simulink model "psbcompensated"  (Simulink 6.0)
settings: Solver=ode15s  SolverMode=SingleTasking  StartTime=0.0  StopTime=0.4  RelTol=1e-4
InitFcn:
  | powericon('psbinitsys',bdroot);
libraries: powerlib2 x35
settings Model: Creator=patrice  LastModifiedBy=batserve  ExtModeTrigMode=oneshot  ExtModeArmWhenConnect=off  ExtModeAutoUpdateStatusClock=off
settings DataIOCC: ExternalInput=[]  LimitDataPoints=off  SaveOutput=off  SignalLoggingName=sigsOut
settings OptimizationCC: BlockReduction=off  BooleanDataType=off
settings DebuggingCC: AlgebraicLoopMsg=none  CheckExecutionContextPreStartOutputMsg=on  CheckExecutionContextRuntimeOutputMsg=on  SolverPrmCheckMsg=none
settings HardwareCC: TargetUnknown=on
settings RTWCC: TemplateMakefile=grt_unix.tmf

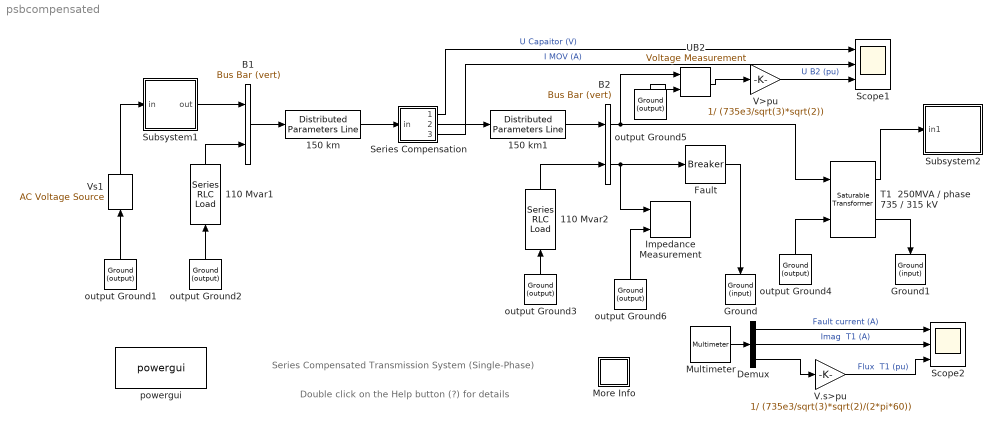
== system psbcompensated ==
  note: Series Compensated Transmission System
      | (Single-Phase)
  note: Double click on the Help button (?) for details
  110 Mvar1 : powerlib2/Elements/Series RLC Load  Tag=PoWeRsYsTeMbLoCk  Orientation=up  a=735000/sqrt(3)  b=60  c=110e6/300  d=110e6  e=0  mesure=None  PSBOutputType=1
  110 Mvar2 : powerlib2/Elements/Series RLC Load  Tag=PoWeRsYsTeMbLoCk  Orientation=up  a=735000/sqrt(3)  b=60  c=110e6/300  d=110e6  e=0  mesure=None  PSBOutputType=1
  150 km : powerlib2/Elements/Distributed Parameters Line  Tag=PoWeRsYsTeMbLoCk  n=1  f=60  r=0.011  l=0.8674e-03  c=13.41e-09  lgt=150  x1=[0 0 0 0; 0.0001244 0 0 0; 0.0002488 0 0 0; 0.0003733 0 0 0; 0.0004977 0 0 0; 0.0006221 0 0 0]  x2=[0 0 0 0; 0.0001244 0 0 0; 0.0002488 0 0 0; 0.0003733 0 0 0; 0.0004977 0 0 0; 0.0006221 0 0 0]  x3=[0 0 0 0; 0.0001244 0 0 0; 0.0002488 0 0 0; 0.0003733 0 0 0; 0.0004977 0 0 0; 0.0006221 0 0 0]  x4=[0 0 0 0; 0.0001244 0 0 0; 0.0002488 0 0 0; 0.0003733 0 0 0; 0.0004977 0 0 0; 0.0006221 0 0 0]  x5=0  mesure=None  PSBOutputType=111111111111111111111111111111
  150 km1 : powerlib2/Elements/Distributed Parameters Line  Tag=PoWeRsYsTeMbLoCk  n=1  f=60  r=0.011  l=0.8674e-03  c=13.41e-09  lgt=150  x1=[0 0 0 0; 0.0001244 0 0 0; 0.0002488 0 0 0; 0.0003733 0 0 0; 0.0004977 0 0 0; 0.0006221 0 0 0]  x2=[0 0 0 0; 0.0001244 0 0 0; 0.0002488 0 0 0; 0.0003733 0 0 0; 0.0004977 0 0 0; 0.0006221 0 0 0]  x3=[0 0 0 0; 0.0001244 0 0 0; 0.0002488 0 0 0; 0.0003733 0 0 0; 0.0004977 0 0 0; 0.0006221 0 0 0]  x4=[0 0 0 0; 0.0001244 0 0 0; 0.0002488 0 0 0; 0.0003733 0 0 0; 0.0004977 0 0 0; 0.0006221 0 0 0]  x5=0  mesure=None  PSBOutputType=111111111111111111111111111111
  B1 : powerlib2/Connectors/Bus Bar (vert)  Tag=PoWeRsYsTeMbLoCk  entrees=2  sorties=1  PSBOutputType=11111111111111111111111111111111111111111111111111111111111111111111111111111111111111111
  B2 : powerlib2/Connectors/Bus Bar (vert)  Tag=PoWeRsYsTeMbLoCk  entrees=2  sorties=2  PSBOutputType=11111111111111111111111111111111111111111111111111111111111111111111111111111111111111111
  Demux : Demux  Outputs=3
  Fault : powerlib2/Elements/Breaker  Tag=PoWeRsYsTeMbLoCk  a=0.01  c=0  rs=inf  cs=0  times="[ 3/60  9/60 ]"  Ts=0  comext=off  mesure=Branch current  PSBOutputType=1
  Ground : powerlib2/Connectors/Ground (input)  Tag=PoWeRsYsTeMbLoCk  Orientation=down
  Ground1 : powerlib2/Connectors/Ground (input)  Tag=PoWeRsYsTeMbLoCk  Orientation=down
  Impedance Measurement : powerlib2/Measurements/Impedance Measurement  Tag=PoWeRsYsTeMbLoCk  kz=1
  More Info : Subsystem
      mask Display: disp('?')
  Multimeter : powerlib2/Measurements/Multimeter  Tag=PoWeRsYsTeMmEaSuReMeNt  PhasorSimulation=off  OutputType=Magnitude  sel=[1 2 3]  L=3  Gain=[1 1 1]  yselected="{'Ib: Fault','Imag: T1  250MVA // phase  735 // 315 kV','Flux: T1  250MVA // phase  735 // 315 kV'};"  PSBOutputType=1  PSBequivalent=0  AxesSetting=[0,0.1,-100,100]  Display=0  SavedBlockNames={}
  Scope1 : Scope  NumInputPorts=3
      settings: DeleteFcn=simscope BlockIsBeingDestroyed  PostSaveFcn=simscope Save  TimeRange=0.4  YMin=-300000~-7500~-1.5  YMax=300000~7500~1.5  DataFormat=Array  MaxDataPoints=100000000
  Scope2 : Scope  NumInputPorts=3
      settings: DeleteFcn=simscope BlockIsBeingDestroyed  PostSaveFcn=simscope Save  TimeRange=0.4  YMin=-10000~-2000~-2  YMax=10000~1000~2  DataFormat=Array  MaxDataPoints=100000000
  Series Compensation : Subsystem
      mask Display: plot(0,0,100,100,[10 40],[50 50], [40 40],[40 60],[60 60],[40 60], [60 90],[50 50])
  Subsystem1 : Subsystem
      mask Display: disp('735 kV\nEquivalent')
  Subsystem2 : Subsystem
      mask Display: disp('315 kV\nEquivalent')
  T1  250MVA / phase  735 / 315 kV : powerlib2/Elements/Saturable Transformer  Tag=PoWeRsYsTeMbLoCk  a=[750e6/3,60]  b=[735000/sqrt(3), 0.001 ,0.15]  c=[315000/sqrt(3), 0.001,0]  w3check=off  d=[315000/sqrt(3), 0.001,0]  e=[0 0 ; 0.0012 1.2; 1.0 1.45 ]  f=[1000]  H=off  matfile='hysteresis'  Initialslope=+1  mesure=Flux and magnetization current ( Imag )  PSBOutputType=1111
  UB2 : powerlib2/Measurements/Voltage Measurement  Tag=PoWeRsYsTeMmEaSuReMeNt  PhasorSimulation=off  OutputType=Magnitude  PSBOutputType=0  PSBequivalent=1
  V.s>pu : Gain  Gain=1/ (735e3/sqrt(3)*sqrt(2)/(2*pi*60))  SaturateOnIntegerOverflow=on
  V>pu : Gain  Gain=1/ (735e3/sqrt(3)*sqrt(2))  SaturateOnIntegerOverflow=on
  Vs1 : powerlib2/Electrical Sources/AC Voltage Source  Tag=PoWeRsYsTeMbLoCk  Orientation=up  A=735000/sqrt(3)*sqrt(2)  P=0  F=60  stime=0  mesure=None  PSBOutputType=1
  output Ground{1..6} (6 alike) : powerlib2/Connectors/Ground (output)  Tag=PoWeRsYsTeMbLoCk  Orientation=up  PSBOutputType=1
  powergui : powerlib2/powergui  Frange=0:500  Ylog=off  Xlog=off  save=off  variable=ZData  ZoomFFT=on  StartTime=0.0  cycles=2  DisplayStyle=off  fundamental=60  FreqAxis=off  MaxFrequency=1000  frequencyindice=1  frequencyindicesteady=1  RmsSteady=1  display=off  Ts=0  methode=off  frequency=60  echomessages=off
  wires:
  T1  250MVA / phase  735 / 315 kV/2 -> Ground1/1
  output Ground4/1 -> T1  250MVA / phase  735 / 315 kV/2
  output Ground5/1 -> UB2/2
  Fault/1 -> Ground/1
  B1/1 -> 150 km/1
  output Ground2/1 -> 110 Mvar1/1
  110 Mvar1/1 -> B1/2
  output Ground1/1 -> Vs1/1
  Vs1/1 -> Subsystem1/1(in)
  Subsystem1/1(out) -> B1/1
  Series Compensation/2(out) -> 150 km1/1
  Series Compensation/1(meas_U) -> Scope1/1  "U Capaitor (V)"
  150 km1/1 -> B2/1
  output Ground3/1 -> 110 Mvar2/1
  110 Mvar2/1 -> B2/2
  T1  250MVA / phase  735 / 315 kV/1 -> Subsystem2/1(in1)
  Series Compensation/3(meas_I) -> Scope1/2  "I MOV (A)"
  B2/1 -> T1  250MVA / phase  735 / 315 kV/1, UB2/1
  Multimeter/1 -> Demux/1
  UB2/1 -> V>pu/1
  V>pu/1 -> Scope1/3  "U B2 (pu)"
  B2/2 -> Fault/1, Impedance Measurement/1
  output Ground6/1 -> Impedance Measurement/2
  Demux/3 -> V.s>pu/1
  Demux/1 -> Scope2/1  "Fault current (A)"
  V.s>pu/1 -> Scope2/3  "Flux  T1 (pu)"
  Demux/2 -> Scope2/2  "Imag  T1 (A)"
  150 km/1 -> Series Compensation/1(in)

== system psbcompensated/More Info ==
  note: Demonstration
  note: This demonstration ilustrates frequency-domain and time-domain analysis of
      | a series-compensated  transmission system
  note: Circuit Description
  note: A 735 kV, 300 km  line is used to  transmit power from bus B1 (735 kV equivalent system) to bus B2 (315 kV equivalent).
      | In order to simplify, only one phase of the system has been represented.
      | (A detailed simulation of  a three-phase series compensated network is presented in the demos and explained in the case studies section of the user's manual.)
      |
      |  In order to increase the transmission capacity, the line is series compensated at its center by a capacitor representing 40% of the line reactance.
      | The line is also shunt compensated at both ends by a 330 Mvar shunt reactance (110 Mvar /phase).
      | Open the  Series Compensation subsystem. Notice that the series capacitor is protected by a Metal Oxide Varistor (MOV) simulated by the Surge arrester block.
      | The 250 MVA, 735 kV / 315 kV transformer is a Saturable Transformer block simulating one phase of the three-phase 750 MVA transformer.
      | A  Multimeter block is used to monitor the fault current as well as the  flux and magnetizing current of the transformer.
  note: You will now study the transient performance of this circuit when a 6-cycle fault is applied at bus B2.
      | Fault is simulated by the Breaker block. Switching times are defined in the Breaker block menu (closing at t = 3 cycles and opening at t = 9 cycles).
  note: Start the simulatiom and observe waveforms on the two Scopes.
      | At t = 3 cycles a line-to-ground fault is applied and the fault current reaches 10 kA (trace 1 of Scope2).
      | During the fault, the MOV conducts at every half cycle (trace 2 of Scope1)  and the voltage across the capacitor (trace 1 of Scope1)  is limited to 263 kV.
      | At t = 9 cycles the fault is cleared. The 15 Hz mode is clearly seen on the capacitor voltage (trace 1 of Scope1) and bus B2 voltage (trace 3 of Scope1).
      | During fault the flux in the transformer is trapped to around 1 pu. At fault clearing  the flux offset and 15 Hz component cause transformer
      | saturation (flux > 1.2 pu, trace 3 of Scope2), producing magnetizing current pulses (trace 2 of Scope2).
  note: Frequency Analysis
  note: Time Domain Simulation- Fault at Bus B2
  note: In order to understand the transient behavior of this series-compensated network, a frequency analysis is first preformed by measuring the Impedance at bus B2.
      | This  measurement is performed by the Impedance measurement block connected at bus B2.
      | Open the Powergui and in the Tools menu select 'Impedance vs Frequency Mesurement'. Click on Display to compute and display the impedance for the 0 - 500 Hz range.
      | The impedance curves show two main parallel resonances (impedance maxima and phase inversion), corresponding to 15 Hz and 300 Hz modes.
      | The 15 Hz mode is due to a parallel resonance of the series capacitance and the two shunt reactances.
      | The 300 Hz mode is  mainly due to resonance of shunt line capacitance and series reactance of the transmission system.
      | These two modes are likely to be excited at fault clearing.
  note: G. Sybille (Hydro-Quebec)

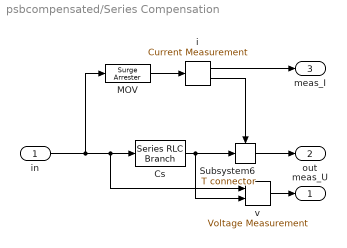
== system psbcompensated/Series Compensation ==
  in : Inport  Port=1  LatchInput=off
  Cs : powerlib2/Elements/Series RLC Branch  Tag=PoWeRsYsTeMbLoCk  a=0  b=0  c=67.6e-6  mesure=None  PSBOutputType=1
  MOV : powerlib2/Elements/Surge Arrester  Tag=PoWeRsYsTeMbLoCk  x1=277e+03  x2=30  x3=500  x4=[.955 50]  x5=[1.0 25]  x6=[.9915 16.5]  mesure=None  PSBOutputType=1
  Subsystem6 : powerlib2/Connectors/T connector  Tag=PoWeRsYsTeMbLoCk  PSBOutputType=1
  i : powerlib2/Measurements/Current Measurement  Tag=PoWeRsYsTeMmEaSuReMeNt  PhasorSimulation=off  OutputType=Magnitude  PSBOutputType=01  PSBequivalent=0
  v : powerlib2/Measurements/Voltage Measurement  Tag=PoWeRsYsTeMmEaSuReMeNt  PhasorSimulation=off  OutputType=Magnitude  PSBOutputType=0  PSBequivalent=0
  meas_U : Outport  InitialOutput=0
  out : Outport  Port=2  InitialOutput=0
  meas_I : Outport  Port=3  InitialOutput=0
  wires:
  v/1 -> meas_U/1
  Subsystem6/1 -> out/1
  in/1 -> Cs/1, v/1, MOV/1
  MOV/1 -> i/1
  i/1 -> meas_I/1
  i/2 -> Subsystem6/Enable
  Cs/1 -> Subsystem6/1, v/2

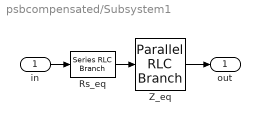
== system psbcompensated/Subsystem1 ==
  in : Inport  Port=1  LatchInput=off
  Rs_eq : powerlib2/Elements/Series RLC Branch  Tag=PoWeRsYsTeMbLoCk  a=2  b=0  c=inf  mesure=None  PSBOutputType=1
  Z_eq : powerlib2/Elements/Parallel RLC Branch  Tag=PoWeRsYsTeMbLoCk  a=180.1  b=.026525  c=117.84e-06  mesure=None  PSBOutputType=1
  out : Outport  InitialOutput=0
  wires:
  Z_eq/1 -> out/1
  in/1 -> Rs_eq/1
  Rs_eq/1 -> Z_eq/1

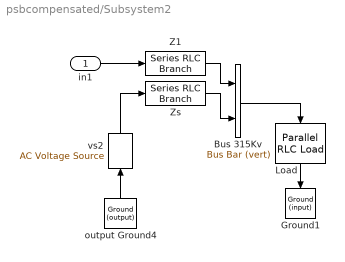
== system psbcompensated/Subsystem2 ==
  in1 : Inport  Port=1  LatchInput=off
  Bus 315Kv : powerlib2/Connectors/Bus Bar (vert)  Tag=PoWeRsYsTeMbLoCk  entrees=2  sorties=1  PSBOutputType=11111111111111111111111111111111111111111111111111111111111111111111111111111111111111111
  Ground1 : powerlib2/Connectors/Ground (input)  Tag=PoWeRsYsTeMbLoCk  Orientation=down
  Load : powerlib2/Elements/Parallel RLC Load  Tag=PoWeRsYsTeMbLoCk  Orientation=down  a=315000/sqrt(3)  b=60  c=200e6  d=0  e=50e6  mesure=None  PSBOutputType=1
  Z1 : powerlib2/Elements/Series RLC Branch  Tag=PoWeRsYsTeMbLoCk  a=0.734  b=0.02085  c=inf  mesure=None  PSBOutputType=1
  Zs : powerlib2/Elements/Series RLC Branch  Tag=PoWeRsYsTeMbLoCk  a=11.0  b=0.2925  c=inf  mesure=None  PSBOutputType=1
  output Ground4 : powerlib2/Connectors/Ground (output)  Tag=PoWeRsYsTeMbLoCk  Orientation=up  PSBOutputType=1
  vs2 : powerlib2/Electrical Sources/AC Voltage Source  Tag=PoWeRsYsTeMbLoCk  Orientation=up  A=315000/sqrt(3)*sqrt(2)  P=20  F=60  stime=0  mesure=None  PSBOutputType=1
  wires:
  Bus 315Kv/1 -> Load/1
  Load/1 -> Ground1/1
  Z1/1 -> Bus 315Kv/1
  Zs/1 -> Bus 315Kv/2
  in1/1 -> Z1/1
  vs2/1 -> Zs/1
  output Ground4/1 -> vs2/1
